simulink model "aaa2"  (R2021b)
settings: Solver=VariableStepAuto  StartTime=0.0  StopTime=20  RelTol=1e-3
libraries: simulink x3
settings Model: Creator=郭义月  LastModifiedBy=郭义月

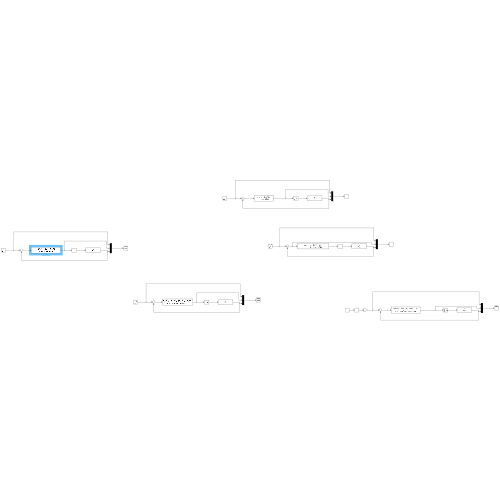
[thumbnail: Simulink's stored preview of the top-level diagram]
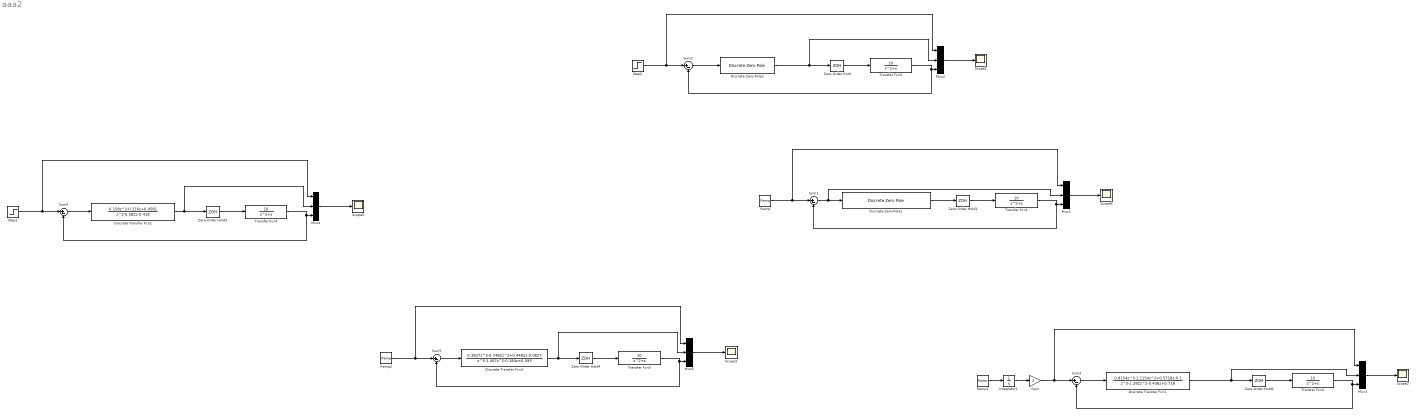
== system aaa2 ==
  Discrete Transfer Fcn1 : DiscreteTransferFcn  Numerator=[0.8154 -1.1154 0.5718 -0.1]  Denominator=[1 -1.282 -0.436 0.718]
  Discrete Transfer Fcn2 : DiscreteTransferFcn  Numerator=[0.158 -0.216 0.0581]  Denominator=[1 -0.582 -0.418]  SampleTime=1
  Discrete Transfer Fcn3 : DiscreteTransferFcn  Numerator=[0.3827 -0.7482 0.4481 -0.0827]  Denominator=[1 -1.407 -0.184 0.593]
  Discrete Zero-Pole1 : DiscreteZeroPole  Zeros=[0.5 0.9]  Poles=[1 -0.718]  Gain=0.5434  SampleTime=-1
  Discrete Zero-Pole2 : DiscreteZeroPole  Zeros=[0.3679]  Poles=[-0.718]  Gain=0.7  SampleTime=-1
  Gain : Gain  Gain=2
  Integrator1 : Integrator
  Mux{1..5} (5 alike) : Mux  Inputs=3
  Ramp : simulink/Sources/Ramp  slope=1  start=0  InitialOutput=0
  Ramp1 : simulink/Sources/Ramp  slope=1  start=0  InitialOutput=0
  Ramp2 : simulink/Sources/Ramp  slope=1  start=0  InitialOutput=0
  Scope{1..3,5..6} (5 alike) : Scope
  Step1 : Step  SampleTime=0
  Step2 : Step  SampleTime=0
  Sum{1..5} (5 alike) : Sum  Inputs=|+-
  Transfer Fcn{1..5} (5 alike) : TransferFcn  Numerator=[10]  Denominator=[1 1 0]
  Zero-Order Hold{,1..4} (5 alike) : ZeroOrderHold  SampleTime=-1
  wires:
  Zero-Order Hold/1 -> Transfer Fcn2/1
  Transfer Fcn2/1 -> Mux2/3, Sum2/2
  Step2/1 -> Mux2/1, Sum2/1
  Mux2/1 -> Scope1/1
  Discrete Zero-Pole2/1 -> Mux2/2, Zero-Order Hold/1
  Sum2/1 -> Discrete Zero-Pole2/1
  Discrete Zero-Pole1/1 -> Zero-Order Hold1/1
  Mux1/1 -> Scope6/1
  Ramp/1 -> Mux1/1, Sum1/1
  Transfer Fcn1/1 -> Mux1/3, Sum1/2
  Sum1/1 -> Mux1/2, Discrete Zero-Pole1/1
  Zero-Order Hold1/1 -> Transfer Fcn1/1
  Zero-Order Hold2/1 -> Transfer Fcn3/1
  Sum3/1 -> Discrete Transfer Fcn1/1
  Discrete Transfer Fcn1/1 -> Mux3/2, Zero-Order Hold2/1
  Transfer Fcn3/1 -> Mux3/3, Sum3/2
  Mux3/1 -> Scope2/1
  Ramp1/1 -> Integrator1/1
  Integrator1/1 -> Gain/1
  Gain/1 -> Mux3/1, Sum3/1
  Discrete Transfer Fcn2/1 -> Zero-Order Hold3/1, Mux4/2
  Mux4/1 -> Scope5/1
  Step1/1 -> Mux4/1, Sum4/1
  Transfer Fcn4/1 -> Mux4/3, Sum4/2
  Sum4/1 -> Discrete Transfer Fcn2/1
  Zero-Order Hold3/1 -> Transfer Fcn4/1
  Discrete Transfer Fcn3/1 -> Zero-Order Hold4/1, Mux5/2
  Sum5/1 -> Discrete Transfer Fcn3/1
  Transfer Fcn5/1 -> Mux5/3, Sum5/2
  Ramp2/1 -> Mux5/1, Sum5/1
  Zero-Order Hold4/1 -> Transfer Fcn5/1
  Mux5/1 -> Scope3/1
